simulink model "Part1"  (R2021b)
settings: Solver=VariableStepAuto  StartTime=0.0  StopTime=25  RelTol=1e-3
settings Model: Creator=homan  LastModifiedBy=homan

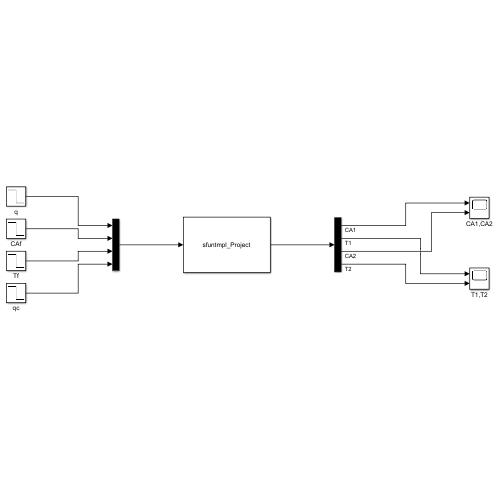
[thumbnail: Simulink's stored preview of the top-level diagram]
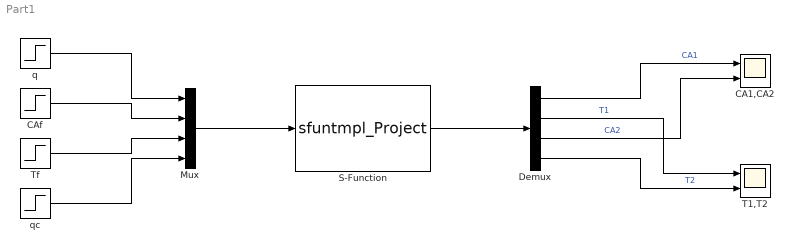
== system Part1 ==
  CA1,CA2 : Scope  NumInputPorts=2
  CAf : Step  Time=5  Before=1  After=1*0.9  SampleTime=0
  Demux : Demux
  Mux : Mux
  S-Function : S-Function  FunctionName=sfuntmpl_Project  SFunctionDeploymentMode=off  EnableBusSupport=off
  T1,T2 : Scope  NumInputPorts=2
  Tf : Step  Time=5  Before=350  After=350*0.9  SampleTime=0
  q : Step  Time=5  Before=100  After=100*0.9  SampleTime=0
  qc : Step  Time=5  Before=99  After=99*0.9  SampleTime=0
  wires:
  qc/1 -> Mux/4
  S-Function/1 -> Demux/1
  Demux/2 -> T1,T2/1  "T1"
  Demux/3 -> CA1,CA2/2  "CA2"
  Tf/1 -> Mux/3
  CAf/1 -> Mux/2
  Demux/1 -> CA1,CA2/1  "CA1"
  Mux/1 -> S-Function/1
  q/1 -> Mux/1
  Demux/4 -> T1,T2/2  "T2"
